simulink model "final_model"  (Simulink 9.2)
settings: Solver=VariableStepAuto  StartTime=0.0  StopTime=250  RelTol=1e-3
values from neighbouring files (symbols this model uses):
  b = 7.66E-5    (= 7.66e-05)    [drone.m]
  d = 5.63E-6    (= 5.63e-06)    [drone.m]
  g = 9.81    [drone.m]
  Ixx = 2.458E-4    (= 0.0002458)    [drone.m]
  Iyy = 4.090E-4    (= 0.000409)    [drone.m]
  Izz = 5.2256E-4    (= 0.00052256)    [drone.m]
  Jr = 5.225E-5    (= 5.225e-05)    [drone.m]
  kd = [20;30;35;2;2;2]    [drone.m]
  kp = [30;25;20;20;20;15]    [drone.m]
  l = 0.135    [drone.m]
  m = 0.494    [drone.m]
  Ts = 0.1    [drone.m]
libraries: simulink x4
settings Model: Creator=Mauri  LastModifiedBy=Mauri
settings Model: SuppressorTable=|
  | <?xml version="1.0" encoding="UTF-8" standalone="yes" ?>
  | <!DOCTYPE boost_serialization>
  | <boost_serialization signature="serialization::archive" version="15">
  | <DiagnosticSuppressor class_id="0" tracking_level="0" version="6">
  | 	<Table class_id="1" tracking_level="0" version="0">
  | 		<count>4</count>
  | 		<bucket_count>8</bucket_count>
  | 		<item_version>0</item_version>
  | 		<item class_id="2" tracking_level="0" version="0">
  | 			<first class_id="3" tracking_level="0" version="6">
  | 				<Source class_id="4" tracking_level="0" version="0">
  | 					<count>1</count>
  | 					<item_version>0</item_version>
  | 					<item>final_model/Ref_yaw1/LimitedCounter</item>
  | 				</Source>
  | 			</first>
  | 			<second class_id="5" tracking_level="0" version="6">
  | 				<SuppressedData class_id="6" tracking_level="0" version="0">
  | 					<count>2</count>
  | 					<bucket_count>8</bucket_count>
  | 					<item_version>0</item_version>
  | 					<item class_id="7" tracking_level="0" version="0">
  | 						<first class_id="8" tracking_level="0" version="6">
  | 							<ID>SimulinkFixedPoint:util:Overflowoccurred</ID>
  | 							<Cause>
  | 								<Source>
  | 									<count>0</count>
  | 									<item_version>0</item_version>
  | 								</Source>
  | 							</Cause>
  | 						</first>
  | 						<second class_id="9" tracking_level="0" version="6">
  | 							<Comment></Comment>
  | 							<User></User>
  | 							<LastModified class_id="10" tracking_level="0" version="0">
  | 								<ptime_date class_id="11" tracking_level="0" version="0">
  | 									<date>20160608</date>
  | 								</ptime_date>
  | 								<ptime_time_duration class_id="12" tracking_level="0" version="0">
  | 									<is_special>0</is_special>
  | 									<time_duration_hours>15</time_duration_hours>
  | 									<time_duration_minutes>23</time_duration_minutes>
  | 									<time_duration_seconds>17</time_duration_seconds>
  | 									<time_duration_fractional_seconds>0</time_duration_fractional_seconds>
  | 								</ptime_time_duration>
  | 							</LastModified>
  | 							<SuppressionType>1</SuppressionType>
  | 						</second>
  | 					</item>
  | 					<item>
  | 						<first>
  | 							<ID>Simulink:DataType:WarningOverFlowDetected</ID>
  | 							<Cause>
  | 								<Source>
  | 									<count>0</count>
  | 									<item_version>0</item_version>
  | 								</Source>
  | 							</Cause>
  | 						</first>
  | 						<second>
  | 							<Comment></Comment>
  | 							<User></User>
  | 							<LastModified>
  | 								<ptime_date>
  | 									<date>20160608</date>
  | 								</ptime_date>
  | 								<ptime_time_duration>
  | 									<is_special>0</is_special>
  | 									<time_duration_hours>15</time_duration_hours>
  | 									<time_duration_minutes>23</time_duration_minutes>
  | 									<time_duration_seconds>17</time_duration_seconds>
  | 									<time_duration_fractional_seconds>0</time_duration_fractional_seconds>
  | 								</ptime_time_duration>
  | 							</LastModified>
  | 							<SuppressionType>1</SuppressionType>
  | 						</second>
  | 					</item>
  | 				</SuppressedData>
  | 			</second>
  | 		</item>
  | 		<item>
  | 			<first>
  | 				<Source>
  | 					<count>1</count>
  | 					<item_version>0</item_version>
  | 					<item>final_model/Ref_x1/LimitedCounter</item>
  | 				</Source>
  | 			</first>
  | 			<second>
  | 				<SuppressedData>
  | 					<count>2</count>
  | 					<bucket_count>8</bucket_count>
  | 					<item_version>0</item_version>
  | 					<item>
  | 						<first>
  | 							<ID>SimulinkFixedPoint:util:Overflowoccurred</ID>
  | 							<Cause>
  | 								<Source>
  | 									<count>0</count>
  | 									<item_version>0</item_version>
  | 								</Source>
  | 							</Cause>
  | 						</first>
  | 						<second>
  | 							<Comment></Comment>
  | 							<User></User>
  | 							<LastModified>
  | 								<ptime_date>
  | 									<date>20160608</date>
  | 								</ptime_date>
  | 								<ptime_time_duration>
  | 									<is_special>0</is_special>
  | 									<time_duration_hours>15</time_duration_hours>
  | 									<time_duration_minutes>23</time_duration_minutes>
  | 									<time_duration_seconds>17</time_duration_seconds>
  | 									<time_duration_fractional_seconds>0</time_duration_fractional_seconds>
  | 								</ptime_time_duration>
  | 							</LastModified>
  | 							<SuppressionType>1</SuppressionType>
  | 						</second>
  | 					</item>
  | 					<item>
  | 						<first>
  | 							<ID>Simulink:DataType:WarningOverFlowDetected</ID>
  | 							<Cause>
  | 								<Source>
  | 									<count>0</count>
  | 									<item_version>0</item_version>
  | 								</Source>
  | 							</Cause>
  | 						</first>
  | 						<second>
  | 							<Comment></Comment>
  | 							<User></User>
  | 							<LastModified>
  | 								<ptime_date>
  | 									<date>20160608</date>
  | 								</ptime_date>
  | 								<ptime_time_duration>
  | 									<is_special>0</is_special>
  | 									<time_duration_hours>15</time_duration_hours>
  | 									<time_duration_minutes>23</time_duration_minutes>
  | 									<time_duration_seconds>17</time_duration_seconds>
  | 									<time_duration_fractional_seconds>0</time_duration_fractional_seconds>
  | 								</ptime_time_duration>
  | 							</LastModified>
  | 							<SuppressionType>1</SuppressionType>
  | 						</second>
  | 					</item>
  | 				</SuppressedData>
  | 			</second>
  | 		</item>
  | 		<item>
  | 			<first>
  | 				<Source>
  | 					<count>1</count>
  | 					<item_version>0</item_version>
  | 					<item>final_model/Ref_y1/LimitedCounter</item>
  | 				</Source>
  | 			</first>
  | 			<second>
  | 				<SuppressedData>
  | 					<count>2</count>
  | 					<bucket_count>8</bucket_count>
  | 					<item_version>0</item_version>
  | 					<item>
  | 						<first>
  | 							<ID>SimulinkFixedPoint:util:Overflowoccurred</ID>
  | 							<Cause>
  | 								<Source>
  | 									<count>0</count>
  | 									<item_version>0</item_version>
  | 								</Source>
  | 							</Cause>
  | 						</first>
  | 						<second>
  | 							<Comment></Comment>
  | 							<User></User>
  | 							<LastModified>
  | 								<ptime_date>
  | 									<date>20160608</date>
  | 								</ptime_date>
  | 								<ptime_time_duration>
  | 									<is_special>0</is_special>
  | 									<time_duration_hours>15</time_duration_hours>
  | 									<time_duration_minutes>23</time_duration_minutes>
  | 									<time_duration_seconds>17</time_duration_seconds>
  | 									<time_duration_fractional_seconds>0</time_duration_fractional_seconds>
  | 								</ptime_time_duration>
  | 							</LastModified>
  | 							<SuppressionType>1</SuppressionType>
  | 						</second>
  | 					</item>
  | 					<item>
  | 						<first>
  | 							<ID>Simulink:DataType:WarningOverFlowDetected</ID>
  | 							<Cause>
  | 								<Source>
  | 									<count>0</count>
  | 									<item_version>0</item_version>
  | 								</Source>
  | 							</Cause>
  | 						</first>
  | 						<second>
  | 							<Comment></Comment>
  | 							<User></User>
  | 							<LastModified>
  | 								<ptime_date>
  | 									<date>20160608</date>
  | 								</ptime_date>
  | 								<ptime_time_duration>
  | 									<is_special>0</is_special>
  | 									<time_duration_hours>15</time_duration_hours>
  | 									<time_duration_minutes>23</time_duration_minutes>
  | 									<time_duration_seconds>17</time_duration_seconds>
  | 									<time_duration_fractional_seconds>0</time_duration_fractional_seconds>
  | 								</ptime_time_duration>
  | 							</LastModified>
  | 							<SuppressionType>1</SuppressionType>
  | 						</second>
  | 					</item>
  | 				</SuppressedData>
  | 			</second>
  | 		</item>
  | 		<item>
  | 			<first>
  | 				<Source>
  | 					<count>1</count>
  | 					<item_version>0</item_version>
  | 					<item>final_model/Ref_z1/LimitedCounter</item>
  | 				</Source>
  | 			</first>
  | 			<second>
  | 				<SuppressedData>
  | 					<count>2</count>
  | 					<bucket_count>8</bucket_count>
  | 					<item_version>0</item_version>
  | 					<item>
  | 						<first>
  | 							<ID>SimulinkFixedPoint:util:Overflowoccurred</ID>
  | 							<Cause>
  | 								<Source>
  | 									<count>0</count>
  | 									<item_version>0</item_version>
  | 								</Source>
  | 							</Cause>
  | 						</first>
  | 						<second>
  | 							<Comment></Comment>
  | 							<User></User>
  | 							<LastModified>
  | 								<ptime_date>
  | 									<date>20160608</date>
  | 								</ptime_date>
  | 								<ptime_time_duration>
  | 									<is_special>0</is_special>
  | 									<time_duration_hours>15</time_duration_hours>
  | 									<time_duration_minutes>23</time_duration_minutes>
  | 									<time_duration_seconds>17</time_duration_seconds>
  | 									<time_duration_fractional_seconds>0</time_duration_fractional_seconds>
  | 								</ptime_time_duration>
  | 							</LastModified>
  | 							<SuppressionType>1</SuppressionType>
  | 						</second>
  | 					</item>
  | 					<item>
  | 						<first>
  | 							<ID>Simulink:DataType:WarningOverFlowDetected</ID>
  | 							<Cause>
  | 								<Source>
  | 									<count>0</count>
  | 									<item_version>0</item_version>
  | 								</Source>
  | 							</Cause>
  | 						</first>
  | 						<second>
  | 							<Comment></Comment>
  | 							<User></User>
  | 							<LastModified>
  | 								<ptime_date>
  | 									<date>20160608</date>
  | 								</ptime_date>
  | 								<ptime_time_duration>
  | 									<is_special>0</is_special>
  | 									<time_duration_hours>15</time_duration_hours>
  | 									<time_duration_minutes>23</time_duration_minutes>
  | 									<time_duration_seconds>17</time_duration_seconds>
  | 									<time_duration_fractional_seconds>0</time_duration_fractional_seconds>
  | 								</ptime_time_duration>
  | 							</LastModified>
  | 							<SuppressionType>1</SuppressionType>
  | 						</second>
  | 					</item>
  | 				</SuppressedData>
  | 			</second>
  | 		</item>
  | 	</Table>
  | </DiagnosticSuppressor>
  | </boost_serialization>
settings DataIOCC: LimitDataPoints=off  SaveFormat=Dataset  SignalLoggingSaveFormat=Dataset
settings OptimizationCC: LifeSpan=auto
settings DebuggingCC: UnderspecifiedInitializationDetection=Simplified  MergeDetectMultiDrivingBlocksExec=error  FcnCallInpInsideContextMsg=error  StateNameClashWarn=none  SFUnexpectedBacktrackingDiag=error  SFNoUnconditionalDefaultTransitionDiag=error  SFExecutionAtInitializationDiag=warning
settings HardwareCC: ProdBitPerPointer=64  ProdBitPerSizeT=64  ProdBitPerPtrDiffT=64  ProdLargestAtomicFloat=Float  ProdIntDivRoundTo=Zero  ProdEndianess=LittleEndian  ProdWordSize=64  ProdHWDeviceType=Intel->x86-64 (Windows64)
settings ModelReferenceCC: PropagateSignalLabelsOutOfModel=on
settings SFSimCC: SimUseLocalCustomCode=on
settings RTWCC: RTWUseLocalCustomCode=on
settings CodeAppCC: StateflowObjectComments=off
settings GRTTargetCC: TargetLangStandard=C99 (ISO)  GeneratePreprocessorConditionals=Use local settings  CombineOutputUpdateFcns=on  GRTInterface=off
settings ConfigComp: CovMetricSettings=dwe  CovHtmlReporting=off  CovSaveCumulativeToWorkspaceVar=off  CovSaveSingleToWorkspaceVar=off  CovExternalEMLEnable=on

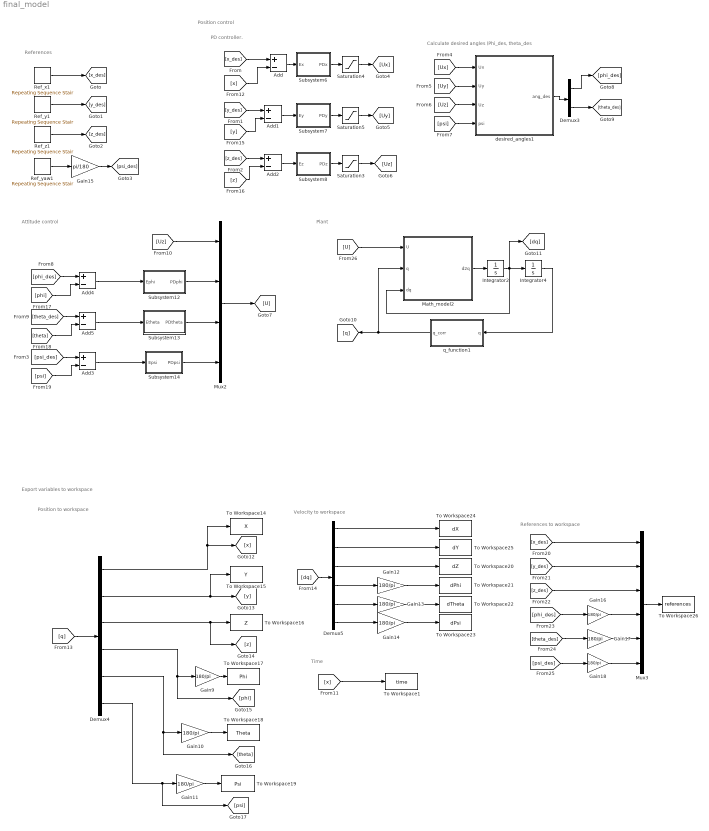
== system final_model ==
  note: Time
  note: Export variables to workspace
  note: Plant
  note: Attitude control
  note: Position control
  note: References
  note: Calculate desired angles (Phi_des, theta_des
  note: PD controller.
  note: Velocity to workspace
  note: Position to workspace
  note: References to workspace
  Add{,1..5} (6 alike) : Sum  Inputs=+-
  Demux3 : Demux  Outputs=2
  Demux4 : Demux  Outputs=6
  Demux5 : Demux  Outputs=6
  Gain{9..14,16..18} (9 alike) : Gain  Gain=180/pi
  Gain15 : Gain  Gain=pi/180
  Integrator2 : Integrator
  Integrator4 : Integrator
  Math_model2 : MATLAB Function  TreatAsAtomicUnit=on
  Mux2 : Mux
  Mux3 : Mux  Inputs=6
  Ref_x1 : simulink/Sources/Repeating Sequence Stair  OutValues=[0 0 0.5 0 -0.5 0 0].'  tsamp=10  OutMin=[]  OutMax=[]  OutDataTypeStr=double  OutputDataTypeScalingMode=double  OutDataType=fixdt(0,8)  ConRadixGroup=Best Precision: Vector-wise  OutScaling=2^-12
  Ref_y1 : simulink/Sources/Repeating Sequence Stair  OutValues=[0 0 0 0.5 0 -0.5 0].'  tsamp=10  OutMin=[]  OutMax=[]  OutDataTypeStr=double  OutputDataTypeScalingMode=double  OutDataType=fixdt(0,8)  ConRadixGroup=Best Precision: Vector-wise  OutScaling=2^-12
  Ref_yaw1 : simulink/Sources/Repeating Sequence Stair  OutValues=[1 1 1 1 1 1 1 2 2 2 2 2 2].'  tsamp=10  OutMin=[]  OutMax=[]  OutDataTypeStr=double  OutputDataTypeScalingMode=double  OutDataType=fixdt(0,8)  ConRadixGroup=Best Precision: Vector-wise  OutScaling=2^-12
  Ref_z1 : simulink/Sources/Repeating Sequence Stair  OutValues=[0 1 1 1 1 1 1 1 0.5 0.5 0.5 0.5 0.5 0.5].'  tsamp=10  OutMin=[]  OutMax=[]  OutDataTypeStr=double  OutputDataTypeScalingMode=double  OutDataType=fixdt(0,8)  ConRadixGroup=Best Precision: Vector-wise  OutScaling=2^-12
  Saturation3 : Saturate  UpperLimit=1000  LowerLimit=0
  Saturation4 : Saturate  UpperLimit=1000  LowerLimit=-1000
  Saturation5 : Saturate  UpperLimit=1000  LowerLimit=-1000
  Subsystem12 : Subsystem
  Subsystem13 : Subsystem
  Subsystem14 : Subsystem
  Subsystem6 : Subsystem
  Subsystem7 : Subsystem
  Subsystem8 : Subsystem
  To Workspace1 : ToWorkspace  VariableName=time  SaveFormat=Timeseries  SampleTime=Ts
  To Workspace14 : ToWorkspace  VariableName=X  SampleTime=Ts
  To Workspace15 : ToWorkspace  VariableName=Y  SampleTime=Ts
  To Workspace16 : ToWorkspace  VariableName=Z  SampleTime=Ts
  To Workspace17 : ToWorkspace  VariableName=Phi  SampleTime=Ts
  To Workspace18 : ToWorkspace  VariableName=Theta  SampleTime=Ts
  To Workspace19 : ToWorkspace  VariableName=Psi  SampleTime=Ts
  To Workspace20 : ToWorkspace  VariableName=dZ  SampleTime=Ts
  To Workspace21 : ToWorkspace  VariableName=dPhi  SampleTime=Ts
  To Workspace22 : ToWorkspace  VariableName=dTheta  SampleTime=Ts
  To Workspace23 : ToWorkspace  VariableName=dPsi  SampleTime=Ts
  To Workspace24 : ToWorkspace  VariableName=dX  SampleTime=Ts
  To Workspace25 : ToWorkspace  VariableName=dY  SampleTime=Ts
  To Workspace26 : ToWorkspace  VariableName=references  SampleTime=Ts
  desired_angles1 : MATLAB Function  TreatAsAtomicUnit=on
  q_function1 : MATLAB Function  TreatAsAtomicUnit=on
  wires:
  Ref_z1/1 -> [z_des]
  Ref_y1/1 -> [y_des]
  Ref_x1/1 -> [x_des]
  Ref_yaw1/1 -> Gain15/1
  Gain15/1 -> [psi_des]
  [Uz] -> desired_angles1/3(Uz)
  [Ux] -> desired_angles1/1(Ux)
  desired_angles1/1(ang_des) -> Demux3/1
  [Uy] -> desired_angles1/2(Uy)
  [z_des] -> Add2/1
  Demux3/2 -> [theta_des]
  Saturation5/1 -> [Uy]
  [y] -> Add1/2
  Add1/1 -> Subsystem7/1(Ey)
  [y_des] -> Add1/1
  [x_des] -> Add/1
  [psi] -> desired_angles1/4(psi)
  Saturation4/1 -> [Ux]
  Subsystem8/1(PDz) -> Saturation3/1
  Demux3/1 -> [phi_des]
  [z] -> Add2/2
  Add2/1 -> Subsystem8/1(Ez)
  [x] -> Add/2
  Subsystem6/1(PDx) -> Saturation4/1
  Subsystem7/1("PDy ") -> Saturation5/1
  Saturation3/1 -> [Uz]
  Add/1 -> Subsystem6/1(Ex)
  Subsystem12/1(PDphi) -> Mux2/2
  [phi] -> Add4/2
  [psi_des] -> Add3/1
  [psi] -> Add3/2
  [theta_des] -> Add5/1
  Subsystem13/1(PDtheta) -> Mux2/3
  Add5/1 -> Subsystem13/1(Etheta)
  Add3/1 -> Subsystem14/1(Epsi)
  [theta] -> Add5/2
  [Uz] -> Mux2/1
  Add4/1 -> Subsystem12/1(Ephi)
  Mux2/1 -> [U]
  Subsystem14/1(PDpsi) -> Mux2/4
  [phi_des] -> Add4/1
  [U] -> Math_model2/1(U)
  q_function1/1(q_corr) -> [q], Math_model2/2(q)
  Integrator4/1 -> q_function1/1(q)
  [q] -> Demux4/1
  Demux4/2 -> To Workspace15/1, [y]
  Demux5/5 -> Gain13/1
  Gain14/1 -> To Workspace23/1
  Demux5/6 -> Gain14/1
  Demux4/1 -> To Workspace14/1, [x]
  Gain12/1 -> To Workspace21/1
  [x_des] -> Mux3/1
  Demux5/4 -> Gain12/1
  Gain17/1 -> Mux3/5
  Gain18/1 -> Mux3/6
  [y_des] -> Mux3/2
  Demux5/2 -> To Workspace25/1
  Mux3/1 -> To Workspace26/1
  Demux4/3 -> [z], To Workspace16/1
  Demux4/6 -> Gain11/1, [psi]
  [phi_des] -> Gain16/1
  [z_des] -> Mux3/3
  Demux4/5 -> Gain10/1, [theta]
  Gain13/1 -> To Workspace22/1
  Demux5/1 -> To Workspace24/1
  Gain9/1 -> To Workspace17/1
  Gain16/1 -> Mux3/4
  [dq] -> Demux5/1
  [psi_des] -> Gain18/1
  Gain10/1 -> To Workspace18/1
  Gain11/1 -> To Workspace19/1
  [theta_des] -> Gain17/1
  Demux4/4 -> Gain9/1, [phi]
  Demux5/3 -> To Workspace20/1
  Integrator2/1 -> Integrator4/1, [dq], Math_model2/3(dq)
  Math_model2/1(d2q) -> Integrator2/1
  [x] -> To Workspace1/1

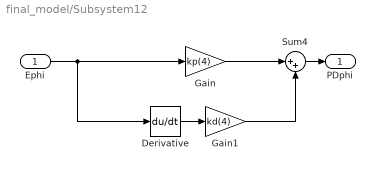
== system final_model/Subsystem12 ==
  Ephi : Inport
  Derivative : Derivative  CoefficientInTFapproximation=1
  Gain : Gain  Gain=kp(4)
  Gain1 : Gain  Gain=kd(4)
  Sum4 : Sum  Inputs=|++
  PDphi : Outport
  wires:
  Gain1/1 -> Sum4/2
  Gain/1 -> Sum4/1
  Derivative/1 -> Gain1/1
  Ephi/1 -> Gain/1, Derivative/1
  Sum4/1 -> PDphi/1

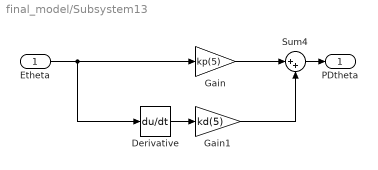
== system final_model/Subsystem13 ==
  Etheta : Inport
  Derivative : Derivative  CoefficientInTFapproximation=1
  Gain : Gain  Gain=kp(5)
  Gain1 : Gain  Gain=kd(5)
  Sum4 : Sum  Inputs=|++
  PDtheta : Outport
  wires:
  Gain1/1 -> Sum4/2
  Sum4/1 -> PDtheta/1
  Etheta/1 -> Gain/1, Derivative/1
  Derivative/1 -> Gain1/1
  Gain/1 -> Sum4/1

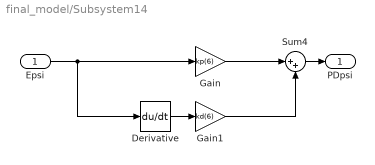
== system final_model/Subsystem14 ==
  Epsi : Inport
  Derivative : Derivative  CoefficientInTFapproximation=1
  Gain : Gain  Gain=kp(6)
  Gain1 : Gain  Gain=kd(6)
  Sum4 : Sum  Inputs=|++
  PDpsi : Outport
  wires:
  Gain1/1 -> Sum4/2
  Gain/1 -> Sum4/1
  Derivative/1 -> Gain1/1
  Epsi/1 -> Gain/1, Derivative/1
  Sum4/1 -> PDpsi/1

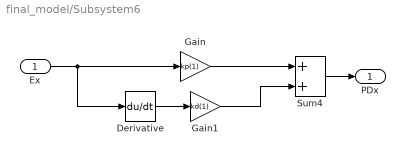
== system final_model/Subsystem6 ==
  Ex : Inport
  Derivative : Derivative  CoefficientInTFapproximation=1
  Gain : Gain  Gain=kp(1)
  Gain1 : Gain  Gain=kd(1)
  Sum4 : Sum
  PDx : Outport
  wires:
  Gain/1 -> Sum4/1
  Ex/1 -> Derivative/1, Gain/1
  Sum4/1 -> PDx/1
  Derivative/1 -> Gain1/1
  Gain1/1 -> Sum4/2

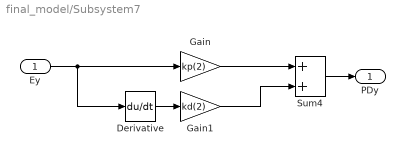
== system final_model/Subsystem7 ==
  Ey : Inport
  Derivative : Derivative  CoefficientInTFapproximation=1
  Gain : Gain  Gain=kp(2)
  Gain1 : Gain  Gain=kd(2)
  Sum4 : Sum
  "PDy " : Outport
  wires:
  Gain1/1 -> Sum4/2
  Derivative/1 -> Gain1/1
  Sum4/1 -> "PDy "/1
  Ey/1 -> Gain/1, Derivative/1
  Gain/1 -> Sum4/1

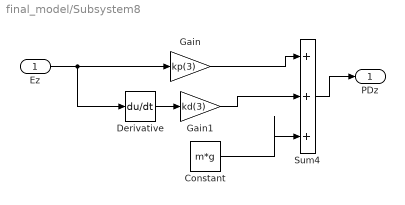
== system final_model/Subsystem8 ==
  Ez : Inport
  Constant : Constant  Value=m*g
  Derivative : Derivative  CoefficientInTFapproximation=1
  Gain : Gain  Gain=kp(3)
  Gain1 : Gain  Gain=kd(3)
  Sum4 : Sum  Inputs=|+++|
  PDz : Outport
  wires:
  Constant/1 -> Sum4/3
  Gain1/1 -> Sum4/2
  Derivative/1 -> Gain1/1
  Sum4/1 -> PDz/1
  Ez/1 -> Gain/1, Derivative/1
  Gain/1 -> Sum4/1

== matlab function Math_model2 ==
  data: U input double size=4,1; q input double size=6,1; dq input double size=6,1; m parameter double; g parameter double; Jr parameter double; Ixx parameter double; Iyy parameter double; Izz parameter double; d2q output double size=6,1; l parameter double; b parameter double; d parameter double
function d2q = model(U,q,dq, m, g, Jr, Ixx, Iyy, Izz,l, b, d)
%% Drone's Math model considering the Equations of Newton-Euler.
% Constants:
%   
%   m: Drone's mass
%   g: Gravity force
%   Jr: Rotor's moment of inertia
%   Ixx: Drone's moment of inertia about axis x
%   Iyy: Drone's moment of inertia about axis y
%   Izz: Drone's moment of inertia about axis z
%   b: Trust constant.
%   d: Drug coefficient.
% Inputs: 
% Control signals
%       U1: z attitude control.
%       U2: roll pid control.
%       U3: pitch pid control.
%       U4: yaw pid control.
% Outputs:
%       q(1): x earth frame position.
%       q(2): y earth frame position.
%       q(3): z earth frame position.
%       q(4): roll angle.
%       q(5): pitch angle.
%       q(6): yaw angle.

% Angular velocities.
sigma = [0;0;0;0];
M = [b b b b;0 l*b 0 -l*b;-l*b 0 l*b 0;-d d -d d];
sigma2 = M\U;
% sigma(1) = U(1) - U(3) - U(4);
% sigma(2) = U(1) + U(2) + U(4);
% sigma(3) = U(1) + U(3) - U(4);
% sigma(4) = U(1) - U(2) + U(4);

% In case of presenting an imaginary value, angular velocity null.
for i=1:4
    if(sigma2(i)<= 0)
       sigma(i) = 0;
    else
       sigma(i) = sqrt(sigma2(i)); 
    end
end
% Euler angles.
phi = q(4);       % Roll angle.
theta = q(5);     % Pitch angle.
psi = q(6);       % Yaw angle.
% Euler angular velocities.
dphi = dq(4);     
dtheta = dq(5);
dpsi = dq(6);
% Define the forces and torques about body frame.
f = U(1);         % Drone Trust body frame.
sigmaT = sigma(1) - sigma(2) + sigma(3) - sigma(4);                  % Total rotors velocity 

tau = [U(2);U(3);U(4)];                                              % Drone torque body frame
                                  
trotor = [dtheta*Jr*sigmaT;-dphi*Jr*sigmaT;Jr*sigmaT];               % Rotors resultant torque

d2x = (f/m)*(sin(phi)*sin(psi) + cos(phi)*sin(theta)*cos(psi));        % acceleration X earth frame.
d2y = (f/m)*(-sin(phi)*cos(psi) + cos(phi)*sin(theta)*sin(psi));       % acceleration Y earth frame.
d2z = -g + (f/m)*(cos(phi)*cos(theta));                                % acceleration Z earth frame.
d2phi = (1/Ixx)*(tau(1)+trotor(1)-dtheta*dpsi*(Izz-Iyy));            % angular acceleration about x axis
d2theta = (1/Iyy)*(tau(2)+trotor(2)-dphi*dpsi*(Ixx-Izz));            % angular acceleration about y axis.
d2psi = (1/Izz)*(tau(3)+trotor(3)-dphi*dtheta*(Iyy-Ixx));            % angular acceleration about z axis.
d2q = [d2x;d2y;d2z;d2phi;d2theta;d2psi];

== matlab function desired_angles1 ==
  data: Ux input double size=1,1; ang_des output double size=2,1; Uy input double size=1,1; Uz input double size=1,1; psi input double size=1,1
function ang_des = calc_des_angles(Ux,Uy,Uz,psi)
% function to calculate the desired roll and pitch  
accel = sqrt(Ux^2+Uy^2+Uz^2);
a1 = sin(psi)*Ux-cos(psi)*Uy;
if (accel > a1 && accel > 0)
   phi_des = asin(a1/accel);
else   
   phi_des = 0; 
end

a2 = cos(psi)*Ux+sin(psi)*Uy;
if (Uz ==0)
    if(a2 <= 0)
        theta_des = pi;
    else
        theta_des = 0;
    end
else
    theta_des = atan(a2/Uz);
end
if(abs(theta_des) == pi)
    theta_des = 0;
end
ang_des = [phi_des;theta_des];
for i=1:2
    if(abs(ang_des(i)) >= 2*pi)
       ang_des(i) = mod(ang_des(i),2*pi);
    else
       ang_des(i) = ang_des(i);
    end
end
% Limit the angles on the range of [-pi pi]
if(ang_des(i) >= pi)
     ang_des(i) = ang_des(i)-2*pi;
else
    if (ang_des(i) <= -pi)
      ang_des(i) = ang_des(i)+2*pi;
    end
end

== matlab function q_function1 ==
  data: q input double size=6,1; q_corr output double size=6,1
function q_corr = limit_angles(q)
% Euler angles between the range of [-2*pi 2*pi]
q_corr = q;
for i=4:6
   if(abs(q(i)) >= 2*pi)
       q_corr(i) = mod(q(i),2*pi);
   else
       q_corr(i) = q(i);
   end
end
% Limit the angles on the range of [-pi pi]
for i=4:6
   if(q_corr(i) >= pi)
       q_corr(i) = q_corr(i)-2*pi;
   else
     if (q_corr(i) <= -pi)
       q_corr(i) = q_corr(i)+2*pi;
     end
   end  
end
% Limit the high into the range of [0 4m]
if(q(3) < 0)
    q_corr(3) = 0;
else
    if (q(3) >= 100)
        q_corr(3) = 100;
    end
end
